simulink model "omniwheels_purepursuit"  (R2023b)
settings: Solver=VariableStepAuto  StartTime=0.0  StopTime=10.0  RelTol=1e-3
undefined symbols (not defined in the file): sampleTime
libraries: mobileRoboticsLib x3, robotalgslib x1
settings Model: Creator=mihai  LastModifiedBy=mihai

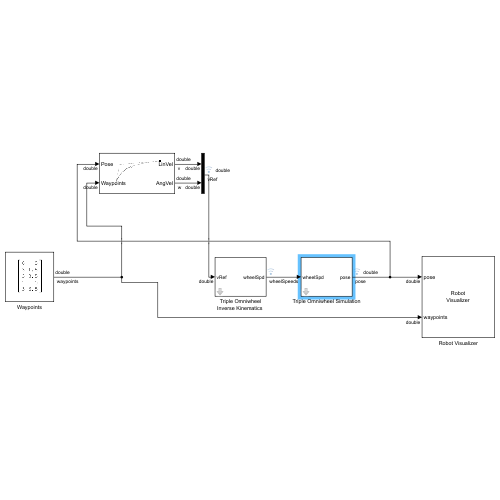
[thumbnail: Simulink's stored preview of the top-level diagram]
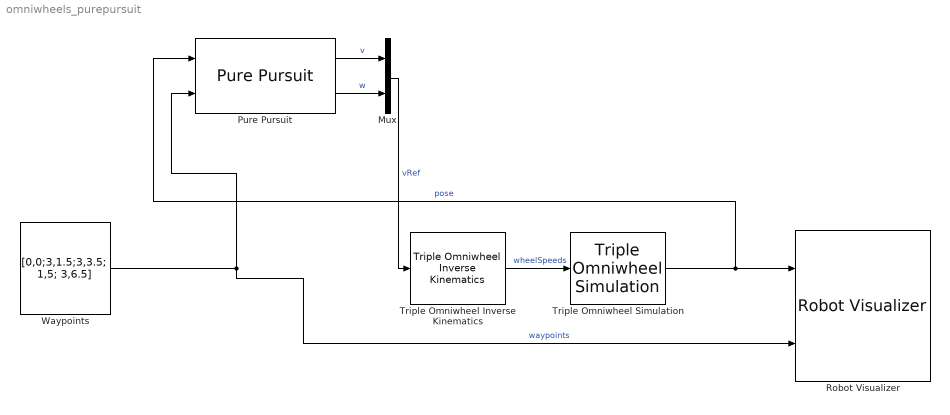
== system omniwheels_purepursuit ==
  Mux : Mux  Inputs=2
  Pure Pursuit : robotalgslib/Pure Pursuit  DesiredLinearVelocity=0.2  MaxAngularVelocity=0.75  LookaheadDistance=0.3  TargetDirPort=off  SimulateUsing=Interpreted execution
  Robot Visualizer : mobileRoboticsLib/Environments/Robot Visualizer  Priority=99  robotRadius=0  showTrajectory=on  hasWaypoints=on  hasLidar=off  sensorOffset=[ 0 0 ]  scanAngles=0  hasObjDetector=off  objDetectorOffset=[ 0, 0 ]  objDetectorAngle=0  objDetectorFOV=0  objDetectorMaxRange=0  objectColors=0  objectMarkers=s
  "Triple Omniwheel Inverse Kinematics " : mobileRoboticsLib/Kinematic Models/Triple Omniwheel/Triple Omniwheel Inverse Kinematics   wheelRadius=wheelRadius  robotRadius=robotRadius  wheelAngles=wheelAngles
      settings: SourceProductName=Mobile Robotics Simulation Toolbox
  Triple Omniwheel Simulation : mobileRoboticsLib/Kinematic Models/Triple Omniwheel/Triple Omniwheel Simulation  wheelRadius=wheelRadius  robotRadius=robotRadius  wheelAngles=wheelAngles  initX=0  initY=0  initAngle=0  Ts=sampleTime
      settings: SourceProductName=Mobile Robotics Simulation Toolbox
  Waypoints : Constant  Value=[0,0;3,1.5;3,3.5; 1,5; 3,6.5]
  wires:
  Triple Omniwheel Simulation/1 -> Pure Pursuit/1, Robot Visualizer/1  "pose"
  Waypoints/1 -> Robot Visualizer/2, Pure Pursuit/2  "waypoints"
  Pure Pursuit/1 -> Mux/1  "v"
  Pure Pursuit/2 -> Mux/2  "w"
  Mux/1 -> "Triple Omniwheel Inverse Kinematics "/1  "vRef"
  "Triple Omniwheel Inverse Kinematics "/1 -> Triple Omniwheel Simulation/1  "wheelSpeeds"
